simulink model "conversor_DAC"  (R2023b)
settings: Solver=VariableStepAuto  StartTime=0.0  StopTime=10.0  RelTol=1e-3
libraries: simulink x3
settings Model: Creator=Pc  LastModifiedBy=Pc

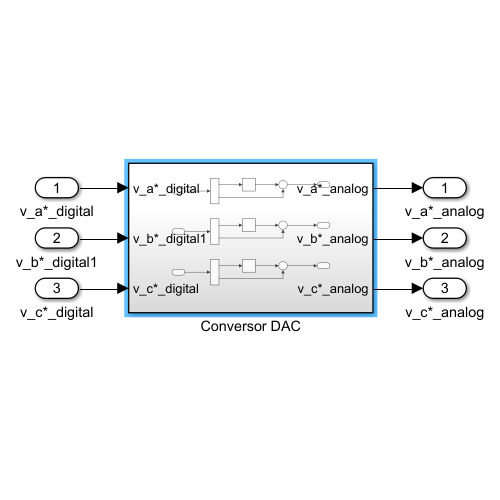
[thumbnail: Simulink's stored preview of the top-level diagram]
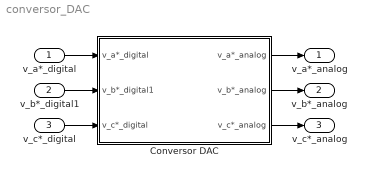
== system conversor_DAC ==
  v_a*_digital : Inport
  v_b*_digital1 : Inport  Port=2
  v_c*_digital : Inport  Port=3
  Conversor DAC : Subsystem
  v_a*_analog : Outport
  v_b*_analog : Outport  Port=2
  v_c*_analog : Outport  Port=3
  wires:
  v_a*_digital/1 -> Conversor DAC/1(v_a*_digital)
  v_b*_digital1/1 -> Conversor DAC/2(v_b*_digital1)
  v_c*_digital/1 -> Conversor DAC/3(v_c*_digital)
  Conversor DAC/1(v_a*_analog) -> v_a*_analog/1
  Conversor DAC/2(v_b*_analog) -> v_b*_analog/1
  Conversor DAC/3(v_c*_analog) -> v_c*_analog/1

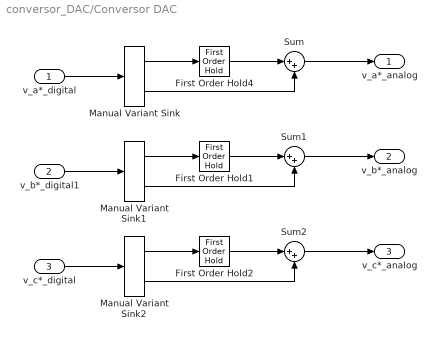
== system conversor_DAC/Conversor DAC ==
  v_a*_digital : Inport
  v_b*_digital1 : Inport  Port=2
  v_c*_digital : Inport  Port=3
  First Order Hold1 : FirstOrderHold  ErrorTolerance=inf  AllowContinuousInput=on
  First Order Hold2 : FirstOrderHold  ErrorTolerance=inf  AllowContinuousInput=on
  First Order Hold4 : FirstOrderHold  ErrorTolerance=inf  AllowContinuousInput=on
  Manual Variant Sink : simulink/Signal Routing/Manual Variant Sink  NumChoices=2  LabelModeActiveChoice=V_2
  Manual Variant Sink1 : simulink/Signal Routing/Manual Variant Sink  NumChoices=2  LabelModeActiveChoice=V_2
  Manual Variant Sink2 : simulink/Signal Routing/Manual Variant Sink  NumChoices=2  LabelModeActiveChoice=V_2
  Sum : Sum  Inputs=|++
  Sum1 : Sum  Inputs=|++
  Sum2 : Sum  Inputs=|++
  v_a*_analog : Outport
  v_b*_analog : Outport  Port=2
  v_c*_analog : Outport  Port=3
  wires:
  Manual Variant Sink/1 -> First Order Hold4/1
  First Order Hold2/1 -> Sum2/1
  Sum1/1 -> v_b*_analog/1
  Manual Variant Sink2/2 -> Sum2/2
  Sum2/1 -> v_c*_analog/1
  Manual Variant Sink1/2 -> Sum1/2
  First Order Hold4/1 -> Sum/1
  Manual Variant Sink2/1 -> First Order Hold2/1
  First Order Hold1/1 -> Sum1/1
  v_c*_digital/1 -> Manual Variant Sink2/1
  v_a*_digital/1 -> Manual Variant Sink/1
  Sum/1 -> v_a*_analog/1
  Manual Variant Sink/2 -> Sum/2
  Manual Variant Sink1/1 -> First Order Hold1/1
  v_b*_digital1/1 -> Manual Variant Sink1/1
